simulink model "phase_estimation"  (R2024a)
settings: Solver=FixedStepAuto  StartTime=0.0  StopTime=Time  FixedStep=0.01  RelTol=1e-3
values from neighbouring files (symbols this model uses):
  rangePost = length(reference)-1    [main.m]
  rangePre = 0    [main.m]
  reference = [traj_ref_x, traj_ref_y,traj_ref_z]    [main.m]
settings Model: Creator=totos  LastModifiedBy=totos

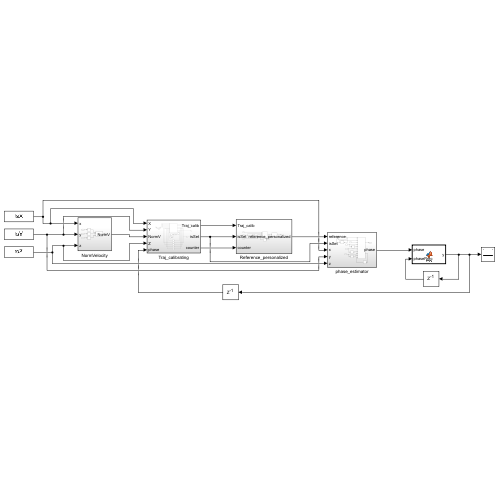
[thumbnail: Simulink's stored preview of the top-level diagram]
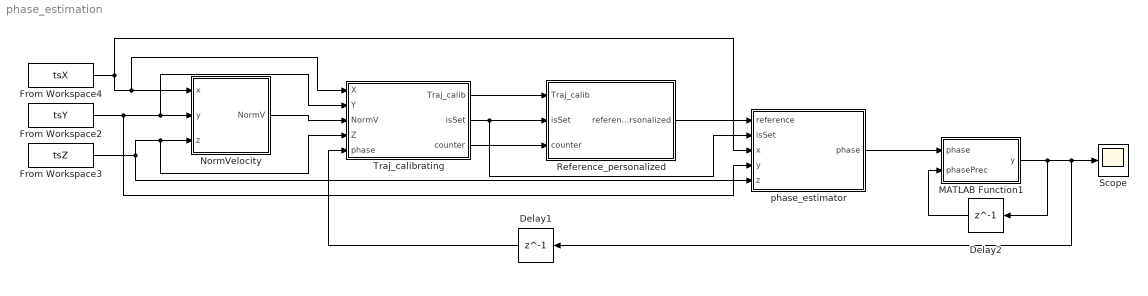
== system phase_estimation ==
  Delay1 : Delay  DelayLength=1
  Delay2 : Delay  DelayLength=1
  From Workspace2 : FromWorkspace  VariableName=tsY
  From Workspace3 : FromWorkspace  VariableName=tsZ
  From Workspace4 : FromWorkspace  VariableName=tsX
  MATLAB Function1 : MATLAB Function  TreatAsAtomicUnit=on
  NormVelocity : Subsystem
  Reference_personalized : Subsystem
  Scope : Scope
  Traj_calibrating : Subsystem
  phase_estimator : Subsystem
  wires:
  From Workspace2/1 -> Traj_calibrating/2(Y), NormVelocity/2(y), phase_estimator/4(y)
  phase_estimator/1(phase) -> MATLAB Function1/1(phase)
  NormVelocity/1(NormV) -> Traj_calibrating/3(NormV)
  Reference_personalized/1(reference_personalized) -> phase_estimator/1(reference)
  Delay1/1 -> Traj_calibrating/5(phase)
  Delay2/1 -> MATLAB Function1/2(phasePrec)
  MATLAB Function1/1(y) -> Scope/1, Delay1/1, Delay2/1
  Traj_calibrating/1(Traj_calib) -> Reference_personalized/1(Traj_calib)
  From Workspace3/1 -> phase_estimator/5(z), Traj_calibrating/4(Z), NormVelocity/3(z)
  From Workspace4/1 -> phase_estimator/3(x), Traj_calibrating/1(X), NormVelocity/1(x)
  Traj_calibrating/3(counter) -> Reference_personalized/3(counter)
  Traj_calibrating/2(isSet) -> phase_estimator/2(isSet), Reference_personalized/2(isSet)

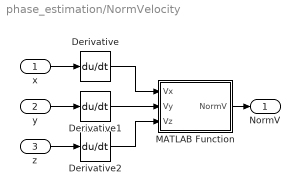
== system phase_estimation/NormVelocity ==
  x : Inport
  y : Inport  Port=2
  z : Inport  Port=3
  Derivative : Derivative
  Derivative1 : Derivative
  Derivative2 : Derivative
  MATLAB Function : MATLAB Function  TreatAsAtomicUnit=on
  NormV : Outport
  wires:
  Derivative2/1 -> MATLAB Function/3(Vz)
  Derivative/1 -> MATLAB Function/1(Vx)
  MATLAB Function/1(NormV) -> NormV/1
  x/1 -> Derivative/1
  Derivative1/1 -> MATLAB Function/2(Vy)
  y/1 -> Derivative1/1
  z/1 -> Derivative2/1

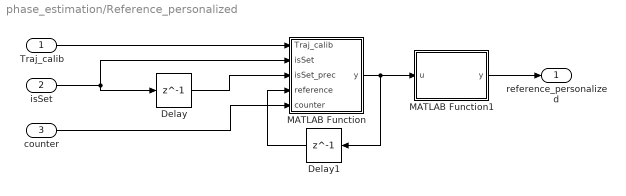
== system phase_estimation/Reference_personalized ==
  Traj_calib : Inport
  isSet : Inport  Port=2
  counter : Inport  Port=3
  Delay : Delay  DelayLength=1
  Delay1 : Delay  DelayLength=1  InitialCondition=reference
  MATLAB Function : MATLAB Function  TreatAsAtomicUnit=on
  MATLAB Function1 : MATLAB Function  TreatAsAtomicUnit=on
  reference_personalized : Outport
  wires:
  Delay1/1 -> MATLAB Function/4(reference)
  Delay/1 -> MATLAB Function/3(isSet_prec)
  MATLAB Function/1(y) -> MATLAB Function1/1(u), Delay1/1
  isSet/1 -> Delay/1, MATLAB Function/2(isSet)
  Traj_calib/1 -> MATLAB Function/1(Traj_calib)
  MATLAB Function1/1(y) -> reference_personalized/1
  counter/1 -> MATLAB Function/5(counter)

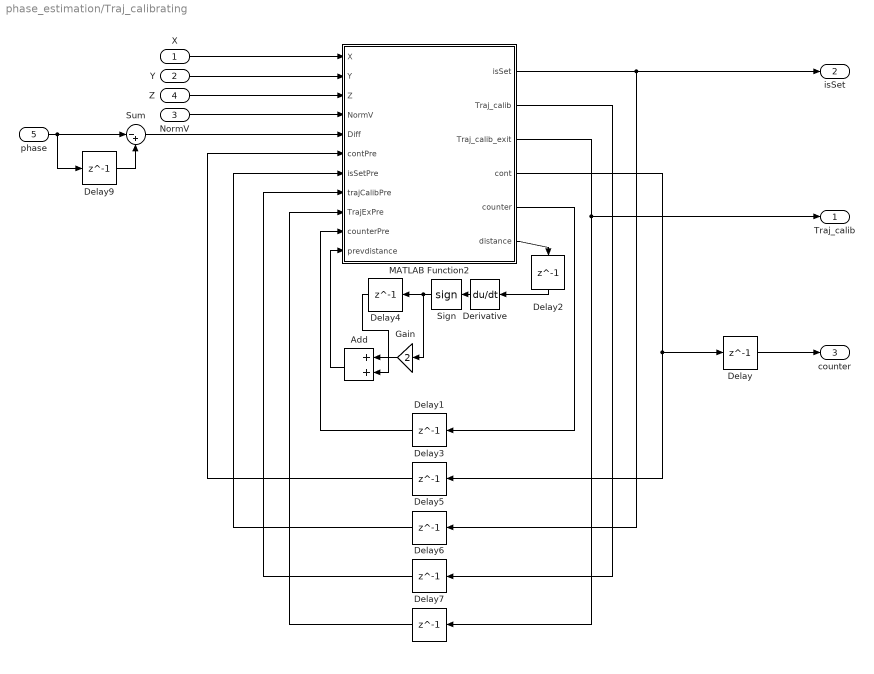
== system phase_estimation/Traj_calibrating ==
  X : Inport
  Y : Inport  Port=2
  NormV : Inport  Port=3
  Z : Inport  Port=4
  phase : Inport  Port=5  PortDimensions=1
  Add : Sum
  Delay{,1..2,4} (4 alike) : Delay  DelayLength=1  InitialCondition=0
  Delay3 : Delay  DelayLength=1
  Delay5 : Delay  DelayLength=1
  Delay6 : Delay  DelayLength=1  InitialCondition=zeros(length(reference)*10,3)
  Delay7 : Delay  DelayLength=1  InitialCondition=zeros(length(reference)*10,3)
  Delay9 : Delay  DelayLength=1
  Derivative : Derivative
  Gain : Gain  Gain=2
  MATLAB Function2 : MATLAB Function  TreatAsAtomicUnit=on
  Sign : Signum
  Sum : Sum  Inputs=|-+
  Traj_calib : Outport
  isSet : Outport  Port=2
  counter : Outport  Port=3
  wires:
  Sum/1 -> MATLAB Function2/5(Diff)
  Delay9/1 -> Sum/2
  MATLAB Function2/3(Traj_calib_exit) -> Delay7/1, Traj_calib/1
  MATLAB Function2/1(isSet) -> Delay5/1, isSet/1
  phase/1 -> Delay9/1, Sum/1
  Delay7/1 -> MATLAB Function2/9(TrajExPre)
  Delay6/1 -> MATLAB Function2/8(trajCalibPre)
  MATLAB Function2/2(Traj_calib) -> Delay6/1
  Delay5/1 -> MATLAB Function2/7(isSetPre)
  Delay3/1 -> MATLAB Function2/6(contPre)
  MATLAB Function2/4(cont) -> Delay/1, Delay3/1
  X/1 -> MATLAB Function2/1(X)
  NormV/1 -> MATLAB Function2/4(NormV)
  Z/1 -> MATLAB Function2/3(Z)
  Y/1 -> MATLAB Function2/2(Y)
  MATLAB Function2/5(counter) -> Delay1/1
  Delay1/1 -> MATLAB Function2/10(counterPre)
  Delay/1 -> counter/1
  MATLAB Function2/6(distance) -> Delay2/1
  Add/1 -> MATLAB Function2/11(prevdistance)
  Derivative/1 -> Sign/1
  Sign/1 -> Delay4/1, Gain/1
  Delay4/1 -> Add/2
  Delay2/1 -> Derivative/1
  Gain/1 -> Add/1

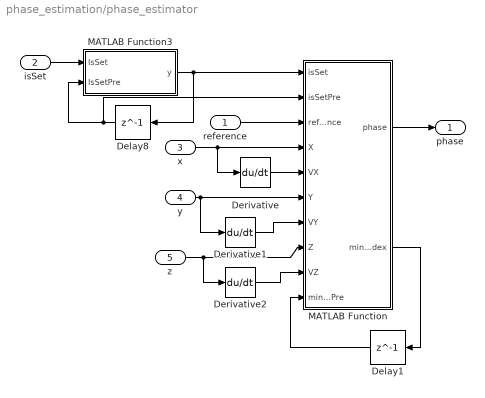
== system phase_estimation/phase_estimator ==
  reference : Inport
  isSet : Inport  Port=2
  x : Inport  Port=3
  y : Inport  Port=4
  z : Inport  Port=5
  Delay1 : Delay  DelayLength=1
  Delay8 : Delay  DelayLength=1
  Derivative : Derivative
  Derivative1 : Derivative
  Derivative2 : Derivative
  MATLAB Function : MATLAB Function  TreatAsAtomicUnit=on
  MATLAB Function3 : MATLAB Function  TreatAsAtomicUnit=on
  phase : Outport  PortDimensions=1
  wires:
  MATLAB Function3/1(y) -> MATLAB Function/1(isSet), Delay8/1
  Delay8/1 -> MATLAB Function3/2(IsSetPre), MATLAB Function/2(isSetPre)
  x/1 -> Derivative/1, MATLAB Function/4(X)
  Derivative1/1 -> MATLAB Function/7(VY)
  z/1 -> Derivative2/1, MATLAB Function/8(Z)
  Derivative/1 -> MATLAB Function/5(VX)
  MATLAB Function/1(phase) -> phase/1
  y/1 -> Derivative1/1, MATLAB Function/6(Y)
  Derivative2/1 -> MATLAB Function/9(VZ)
  isSet/1 -> MATLAB Function3/1(IsSet)
  reference/1 -> MATLAB Function/3(reference)
  MATLAB Function/2(min_index) -> Delay1/1
  Delay1/1 -> MATLAB Function/10(min_index_Pre)

== matlab function phase_estimation/phase_estimator/MATLAB Function3 ==
  data: IsSet input size=1; y output size=1; IsSetPre input size=1
function y = fcn(IsSet, IsSetPre)
if IsSetPre~=2
    y=IsSet;
else
    y=2;
end

== matlab function phase_estimation/MATLAB Function1 ==
  data: phase input; y output; phasePrec input
function y = fcn(phase ,phasePrec)
if(phase-phasePrec)> pi
    y=phasePrec;
else
    y=phase;
end

== matlab function phase_estimation/NormVelocity/MATLAB Function ==
  data: Vx input; NormV output; Vy input; Vz input
function NormV = fcn(Vx,Vy,Vz)
NormV=sqrt(Vx^2+Vy^2+Vz^2);

== matlab function phase_estimation/Reference_personalized/MATLAB Function ==
  settings: updateMethod=DISCRETE  sampleTime=ts
  data: Traj_calib input; y output; isSet input; isSet_prec input; reference input; counter input
function y = fcn(Traj_calib, isSet, isSet_prec, reference, counter)
y=reference;
if(isSet==2&&isSet_prec==1)
    L = length(reference);
    Index=1:counter;
    newIndex=((0:L-1)*(counter-1)/(L-1))+1;
    % Interpolazione per ottenere i nuovi punti
    newX = interp1(Index, Traj_calib(1:counter,1), newIndex);
    newY = interp1(Index, Traj_calib(1:counter,2), newIndex);
    newZ = interp1(Index, Traj_calib(1:counter,3), newIndex);
    res=[newX ; newY; newZ]';
    % Step 1: Traslate
    centroid_traj = mean(res);
    centroid_ref = mean(reference);
    traj_centered = res - centroid_traj;
    P_ref_centered = reference - centroid_ref;
    
    % Step 2: Scale P_ref to match traj
    scale_factors = std(traj_centered) ./ std(P_ref_centered);
    for i=1:length(scale_factors)
        if isnan(scale_factors(i))
            scale_factors(i)=1;
        end
    end
    P_ref_scaled = P_ref_centered .* scale_factors;
    
    % Step 3: Rotate P_ref to match traj
    [U, ~, V] = svd(P_ref_scaled' * traj_centered);
    rotation_matrix = V * U';
    if det(rotation_matrix) < 0
        V(:,end) = -V(:,end);
        rotation_matrix = V * U';
    end
    P_ref_rotated = (rotation_matrix * P_ref_scaled')';
    
    % Step 4: Translate back to the original position
    traj_ref_trasl = P_ref_rotated + centroid_traj;
        for i=1:length(traj_ref_trasl)
            y(i,:)=[traj_ref_trasl(i,:)];
        end
end

== matlab function phase_estimation/Reference_personalized/MATLAB Function1 ==
  data: u input; y output
function y = fcn(u)

y = [u(1:end-1,:) diff(u)];

== matlab function phase_estimation/Traj_calibrating/MATLAB Function2 ==
  data: X input size=1; isSet output size=1; Y input size=1; Z input size=1; NormV input size=1; Diff input size=1; Traj_calib output size=[length(reference)*10 3]; Traj_calib_exit output size=[length(reference)*10 3]; cont output size=1; contPre input size=1; isSetPre input size=1; trajCalibPre input size=[length(reference)*10 3]; TrajExPre input size=[length(reference)*10 3]; epsilon parameter size=1; counter output size=1; counterPre input size=1; distance output; prevdistance input

function [isSet, Traj_calib, Traj_calib_exit,cont,counter,distance] = fcn(X, Y, Z, NormV, Diff, contPre, isSetPre, trajCalibPre, TrajExPre,epsilon,counterPre,prevdistance)
Traj_calib_exit=TrajExPre;
Traj_calib=trajCalibPre;
distance=0;
if isSetPre == 0
    if NormV > epsilon
        isSet = 1;  % Start trajectory calibration
        Traj_calib(1,:) = [X, Y, Z];  % Initialize trajectory with the first point
        cont=contPre+1;
        counter=0;
    else
        isSet = 0;  % Still not started
        cont=contPre;
        counter=0;
    end
elseif isSetPre == 1
    if counterPre==0
            isSet = 1;  % Continue trajectory calibration
            cont=contPre+1;
            Traj_calib(cont,:) = [X, Y, Z];
            counter=0;
            if cont>12
                segment = Traj_calib(cont-9:cont,:);
                distanze = sqrt(sum(([Traj_calib(1:9,:) diff(Traj_calib(1:10,:))]  - [segment(1:9,:) diff(segment)]) .^ 2, 2));
                distance = mean(distanze);
                if(prevdistance==1 )
                    counter=15000;
                    cont=cont-10;
                    isSet = 2;  % Trajectory calibration complete
                    Traj_calib_exit=Traj_calib;
                end
            end
    else
        if counterPre==15000
            cont=contPre;
            counter=15000;
            if Diff >pi
                counter=1;
                Traj_calib(1,:) = [X, Y, Z];
                cont=1;
            end
            isSet=1;
        else
            if Diff >pi
                if counterPre==1 || abs(contPre-counterPre)<counterPre/3
                    counter=contPre;
                    cont=0;
                    isSet = 2;  % Trajectory calibration complete
                    Traj_calib_exit=Traj_calib;
                else
                    counter=counterPre;
                    cont=0;
                    isSet=1;
                end
            else
                counter=counterPre;
                isSet = 1;  % Continue trajectory calibration
                cont=contPre+1;
                Traj_calib(cont,:) = [X, Y, Z];
            end
        end
    end
else
    counter=counterPre;  
    Traj_calib(1,:) = [X, Y, Z];
    cont=1;
    isSet = 1;
end

== matlab function phase_estimation/phase_estimator/MATLAB Function ==
  data: isSet input; isSetPre input; reference input; phase output size=1; X input; VX input; Y input; VY input; Z input; VZ input; min_index output; min_index_Pre input; rangePre parameter; rangePost parameter
function [phase, min_index] = fcn(isSet, isSetPre, reference,X,VX,Y,VY,Z,VZ, min_index_Pre,rangePre,rangePost)
min_index=0;
if isSet==2
    if isSetPre==2
        if min_index_Pre-rangePre<1 && min_index_Pre+rangePost>length(reference)
            ref=reference;
            index=1:length(reference);
        elseif min_index_Pre-rangePre<1
            ref=reference([1:min_index_Pre+rangePost,length(reference)-rangePre+min_index:length(reference)],:);
            index=[1:min_index_Pre+rangePost,length(reference)-rangePre+min_index:length(reference)];
        elseif min_index_Pre+rangePost>length(reference)
            ref=reference([min_index_Pre-rangePre:length(reference),1:min_index_Pre+rangePost-length(reference)],:);
            index=[min_index_Pre-rangePre:length(reference),1:min_index_Pre+rangePost-length(reference)];
        else
            ref=reference(min_index_Pre-rangePre:min_index_Pre+rangePost,:);
            index=min_index_Pre-rangePre:min_index_Pre+rangePost;
        end
        p=[X,Y,Z,VX,VY,VZ];
        distances = sqrt(sum((ref - p) .^ 2, 2));
        [~, index1] = min(distances);
        min_index=index(index1);
        phase=2*pi/length(reference)*min_index;
    else
        p=[X,Y,Z,VX,VY,VZ];
        distances = sqrt(sum((reference - p) .^ 2, 2));
        [~, min_index] = min(distances);
        phase=2*pi/length(reference)*min_index;
    end 
else
    phase=0;
end
